simulink model "cloud9_powerTask"  (R2024b)
settings: Solver=VariableStepAuto  StartTime=0.0  StopTime=10.0  RelTol=1e-3
libraries: spsThreePhaseVIMeasurementLib x6, spsThreePhaseTransformerTwoWindingsLib x5, spsThreePhaseBreakerLib x4, spsThreePhaseSourceLib x3, spsThreePhaseParallelRLCBranchLib x1, sps_lib x1
settings Model: Creator=ASUS  LastModifiedBy=ASUS

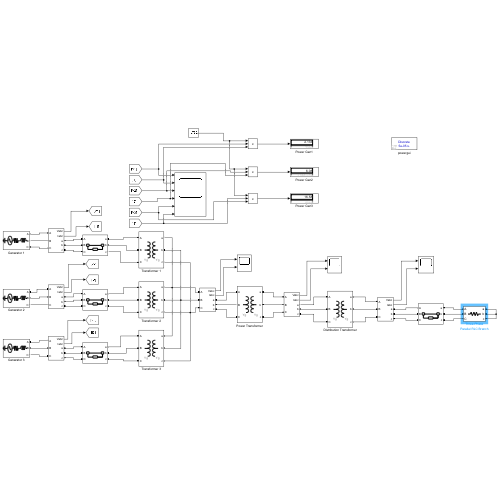
[thumbnail: Simulink's stored preview of the top-level diagram]
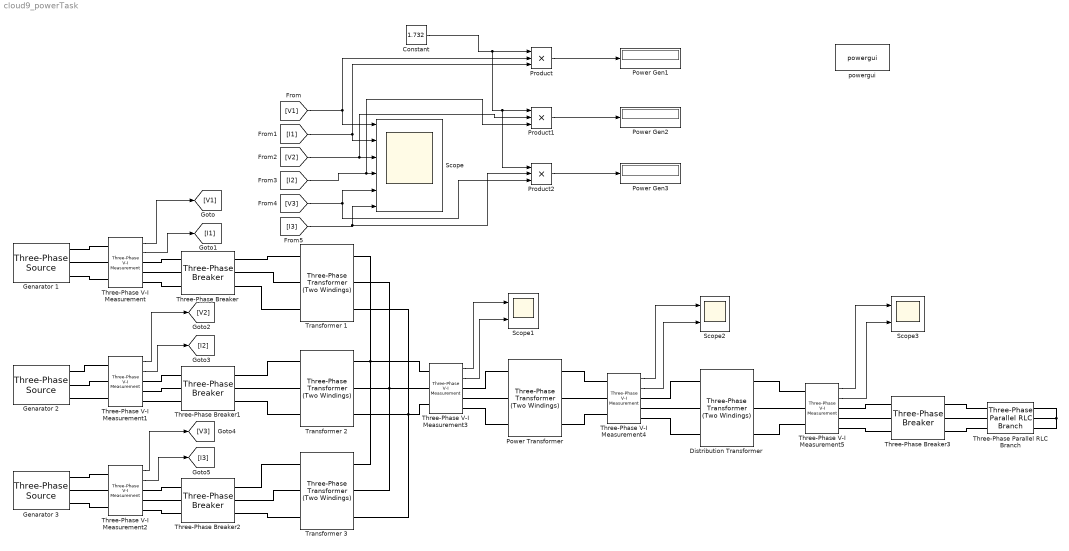
== system cloud9_powerTask ==
  Constant : Constant  Value=1.732
  Distribution Transformer : spsThreePhaseTransformerTwoWindingsLib/Three-Phase Transformer (Two Windings)  Winding1Connection=Yg  Winding2Connection=Yg  CoreType=Three single-phase transformers  SetSaturation=off  Hysteresis=off  DataFile='hysteresis'  SetInitialFlux=off  Measurements=None  UNITS=pu  NominalPower=[ 2e6 , 50 ]  Winding1=[ 11e3 , 0.002 , 0.08 ]  Winding2=[ 0.4e3 , 0.002 , 0.08 ]  Rm=500  Lm=500  L0=0.5  Saturation=[ 0,0 ; 0.0024,1.2 ; 1.0,1.52 ]  InitialFluxes=[ 0.8 , -0.8 , 0.7 ]  BreakLoop=off  DiscreteSolver=Trapezoidal iterative  DataType=off  TransfoNumber=1
  Genarator 1 : spsThreePhaseSourceLib/Three-Phase Source  InternalConnection=Yg  VoltagePhases=off  Voltage=11e3  PhaseAngle=0  Voltage_phases=[25e3 25e3 25e3]/sqrt(3)  PhaseAngles_phases=[0 -120 +120]  Frequency=50  NonIdealSource=on  SpecifyImpedance=off  Resistance=0.8929  Inductance=16.58e-3  ShortCircuitLevel=100e6  BaseVoltage=11e3  XRratio=7  BusType=PV  Pref=1000e3  Qref=0  Prefabc=[10e3, 10e3, 10e3]  Qrefabc=[0, 0, 0]  Qmin=-inf  Qmax=inf
  Genarator 2 : spsThreePhaseSourceLib/Three-Phase Source  InternalConnection=Yg  VoltagePhases=off  Voltage=12e3  PhaseAngle=0  Voltage_phases=[25e3 25e3 25e3]/sqrt(3)  PhaseAngles_phases=[0 -120 +120]  Frequency=50  NonIdealSource=on  SpecifyImpedance=off  Resistance=0.8929  Inductance=16.58e-3  ShortCircuitLevel=100e6  BaseVoltage=12e3  XRratio=7  BusType=PV  Pref=2000e3  Qref=0  Prefabc=[10e3, 10e3, 10e3]  Qrefabc=[0, 0, 0]  Qmin=-inf  Qmax=inf
  Genarator 3 : spsThreePhaseSourceLib/Three-Phase Source  InternalConnection=Yg  VoltagePhases=off  Voltage=10e3  PhaseAngle=0  Voltage_phases=[25e3 25e3 25e3]/sqrt(3)  PhaseAngles_phases=[0 -120 +120]  Frequency=50  NonIdealSource=on  SpecifyImpedance=off  Resistance=0.8929  Inductance=16.58e-3  ShortCircuitLevel=100e6  BaseVoltage=10e3  XRratio=7  BusType=PV  Pref=4000e3  Qref=0  Prefabc=[10e3, 10e3, 10e3]  Qrefabc=[0, 0, 0]  Qmin=-inf  Qmax=inf
  Power Gen1 : Display
  Power Gen2 : Display
  Power Gen3 : Display
  Power Transformer : spsThreePhaseTransformerTwoWindingsLib/Three-Phase Transformer (Two Windings)  Winding1Connection=Yg  Winding2Connection=Yg  CoreType=Three single-phase transformers  SetSaturation=off  Hysteresis=off  DataFile='hysteresis'  SetInitialFlux=off  Measurements=None  UNITS=pu  NominalPower=[ 7e6 , 50 ]  Winding1=[ 132e3 , 0.002 , 0.08 ]  Winding2=[ 11e3 , 0.002 , 0.08 ]  Rm=500  Lm=200  L0=0.5  Saturation=[ 0,0 ; 0.0024,1.2 ; 1.0,1.52 ]  InitialFluxes=[ 0.8 , -0.8 , 0.7 ]  BreakLoop=off  DiscreteSolver=Trapezoidal iterative  DataType=off  TransfoNumber=1
  Product : Product  Inputs=3
  Product1 : Product  Inputs=3
  Product2 : Product  Inputs=3
  Scope : Scope  NumInputPorts=6
  Scope1 : Scope  NumInputPorts=2
  Scope2 : Scope  NumInputPorts=2
  Scope3 : Scope  NumInputPorts=2
  Three-Phase Parallel RLC Branch : spsThreePhaseParallelRLCBranchLib/Three-Phase Parallel RLC Branch  LConnTagsString=A|B|C  RConnTagsString=A|B|C  BranchType=R  Resistance=7000000  Inductance=1e-3  Capacitance=1e-6  Measurements=None
  Three-Phase V-I Measurement{,1..5} (6 alike) : spsThreePhaseVIMeasurementLib/Three-Phase V-I Measurement  VoltageMeasurement=phase-to-ground  SetLabelV=off  LabelV=Vabc  Vpu=off  VpuLL=off  CurrentMeasurement=yes  SetLabelI=off  LabelI=Iabc  Ipu=off  Pbase=100e6  Vbase=500e3  OutputType=Complex  PhasorSimulation=off  PSBequivalent=0
  Three-Phase Breaker{,1..3} (4 alike) : spsThreePhaseBreakerLib/Three-Phase Breaker  InitialState=closed  SwitchA=on  SwitchB=on  SwitchC=on  SwitchTimes="[1/60  5/60]"  External=off  BreakerResistance=0.01  SnubberResistance=1e6  SnubberCapacitance=inf  Measurements=None
  Transformer 1 : spsThreePhaseTransformerTwoWindingsLib/Three-Phase Transformer (Two Windings)  Winding1Connection=Yg  Winding2Connection=Yg  CoreType=Three single-phase transformers  SetSaturation=off  Hysteresis=off  DataFile='hysteresis'  SetInitialFlux=off  Measurements=None  UNITS=pu  NominalPower=[ 1e6 , 50 ]  Winding1=[ 11e3 , 0.002 , 0.08 ]  Winding2=[ 132e3 , 0.002 , 0.08 ]  Rm=500  Lm=200  L0=0.5  Saturation=[ 0,0 ; 0.0024,1.2 ; 1.0,1.52 ]  InitialFluxes=[ 0.8 , -0.8 , 0.7 ]  BreakLoop=off  DiscreteSolver=Trapezoidal iterative  DataType=off  TransfoNumber=1
  Transformer 2 : spsThreePhaseTransformerTwoWindingsLib/Three-Phase Transformer (Two Windings)  Winding1Connection=Yg  Winding2Connection=Yg  CoreType=Three single-phase transformers  SetSaturation=off  Hysteresis=off  DataFile='hysteresis'  SetInitialFlux=off  Measurements=None  UNITS=pu  NominalPower=[ 2e6 , 50 ]  Winding1=[ 12e3 , 0.002 , 0.08 ]  Winding2=[ 132e3 , 0.002 , 0.08 ]  Rm=500  Lm=200  L0=0.5  Saturation=[ 0,0 ; 0.0024,1.2 ; 1.0,1.52 ]  InitialFluxes=[ 0.8 , -0.8 , 0.7 ]  BreakLoop=off  DiscreteSolver=Trapezoidal iterative  DataType=off  TransfoNumber=1
  Transformer 3 : spsThreePhaseTransformerTwoWindingsLib/Three-Phase Transformer (Two Windings)  Winding1Connection=Yg  Winding2Connection=Yg  CoreType=Three single-phase transformers  SetSaturation=off  Hysteresis=off  DataFile='hysteresis'  SetInitialFlux=off  Measurements=None  UNITS=pu  NominalPower=[ 4e6 , 50 ]  Winding1=[ 10e3 , 0.002 , 0.08 ]  Winding2=[ 132e3 , 0.002 , 0.08 ]  Rm=500  Lm=200  L0=0.5  Saturation=[ 0,0 ; 0.0024,1.2 ; 1.0,1.52 ]  InitialFluxes=[ 0.8 , -0.8 , 0.7 ]  BreakLoop=off  DiscreteSolver=Trapezoidal iterative  DataType=off  TransfoNumber=1
  powergui : sps_lib/powergui  Priority=1  SimulationMode=Discrete  SampleTime=50e-6  frequency=60  Iterations=50  frequencyindice=50  Pbase=100e6  ErrMax=1e-4  UnitsV=kV  UnitsW=MW  buscounter=0  FunctionMessages=off  echomessages=off  EnableUseOfTLC=off  CurrentSourceSwitches=off  DisableSnubberDevices=off  DisableRonSwitches=off  DisableVfSwitches=off  DisplayEquations=off  AutomaticDiscreteSolvers=off  SolverType=Tustin/Backward Euler (TBE)  Interpol=off  ExternalGateDelay=off  methode=off  Ts=100  x0status=blocks  SPID=on  SwTol=0  HookPort=off  NonlinearTolerance=1e-4  nMaxIteration=100  ContinueOnMaxIteration=off  RestoreLinks=warning  ResistiveCurrentMeasurement=off  Frange=[0:2:500]  Ylog=off  Xlog=on  ShowGrid=off  save=off  variable=ZData  structure=0  ZoomFFT=off  StartTime=0.0  cycles=1  DisplayStyle=1  fundamental=60  FreqAxis=off  MaxFrequency=1000  frequencyindicesteady=1  RmsSteady=1  display=off
  wires:
  Three-Phase V-I Measurement/1 -> [V1]
  Three-Phase V-I Measurement/2 -> [I1]
  Three-Phase V-I Measurement1/1 -> [V2]
  Three-Phase V-I Measurement1/2 -> [I2]
  Three-Phase V-I Measurement2/1 -> [V3]
  Three-Phase V-I Measurement2/2 -> [I3]
  [V1] -> Scope/1, Product/2
  [I1] -> Product/3, Scope/2
  [V2] -> Product1/2, Scope/3
  [I2] -> Product1/3, Scope/4
  [V3] -> Scope/5, Product2/3
  [I3] -> Product2/2, Scope/6
  Three-Phase V-I Measurement3/1 -> Scope1/1
  Three-Phase V-I Measurement3/2 -> Scope1/2
  Three-Phase V-I Measurement4/1 -> Scope2/1
  Three-Phase V-I Measurement4/2 -> Scope2/2
  Three-Phase V-I Measurement5/1 -> Scope3/1
  Three-Phase V-I Measurement5/2 -> Scope3/2
  Constant/1 -> Product2/1, Product1/1, Product/1
  Product/1 -> Power Gen1/1
  Product1/1 -> Power Gen2/1
  Product2/1 -> Power Gen3/1
  connections:
  Three-Phase Breaker/RConn1 -- Transformer 1/LConn1
  Three-Phase Breaker/RConn2 -- Transformer 1/LConn2
  Three-Phase Breaker/RConn3 -- Transformer 1/LConn3
  Three-Phase Breaker1/RConn1 -- Transformer 2/LConn1
  Three-Phase Breaker1/RConn2 -- Transformer 2/LConn2
  Three-Phase Breaker1/RConn3 -- Transformer 2/LConn3
  Three-Phase Breaker2/RConn1 -- Transformer 3/LConn1
  Three-Phase Breaker2/RConn2 -- Transformer 3/LConn2
  Three-Phase Breaker2/RConn3 -- Transformer 3/LConn3
  Genarator 1/RConn1 -- Three-Phase V-I Measurement/LConn1
  Genarator 1/RConn2 -- Three-Phase V-I Measurement/LConn2
  Genarator 1/RConn3 -- Three-Phase V-I Measurement/LConn3
  Genarator 2/RConn1 -- Three-Phase V-I Measurement1/LConn1
  Genarator 2/RConn2 -- Three-Phase V-I Measurement1/LConn2
  Genarator 2/RConn3 -- Three-Phase V-I Measurement1/LConn3
  Genarator 3/RConn1 -- Three-Phase V-I Measurement2/LConn1
  Genarator 3/RConn2 -- Three-Phase V-I Measurement2/LConn2
  Genarator 3/RConn3 -- Three-Phase V-I Measurement2/LConn3
  Three-Phase V-I Measurement/RConn1 -- Three-Phase Breaker/LConn1
  Three-Phase V-I Measurement/RConn2 -- Three-Phase Breaker/LConn2
  Three-Phase V-I Measurement/RConn3 -- Three-Phase Breaker/LConn3
  Three-Phase V-I Measurement1/RConn1 -- Three-Phase Breaker1/LConn1
  Three-Phase V-I Measurement1/RConn2 -- Three-Phase Breaker1/LConn2
  Three-Phase V-I Measurement1/RConn3 -- Three-Phase Breaker1/LConn3
  Three-Phase V-I Measurement2/RConn1 -- Three-Phase Breaker2/LConn1
  Three-Phase V-I Measurement2/RConn2 -- Three-Phase Breaker2/LConn2
  Three-Phase V-I Measurement2/RConn3 -- Three-Phase Breaker2/LConn3
  Three-Phase V-I Measurement3/LConn1 -- Transformer 3/RConn1 -- Transformer 1/RConn1 -- Transformer 2/RConn1
  Transformer 2/RConn2 -- Transformer 1/RConn2 -- Three-Phase V-I Measurement3/LConn2 -- Transformer 3/RConn2
  Transformer 2/RConn3 -- Transformer 1/RConn3 -- Three-Phase V-I Measurement3/LConn3 -- Transformer 3/RConn3
  Three-Phase V-I Measurement3/RConn1 -- Power Transformer/LConn1
  Three-Phase V-I Measurement3/RConn2 -- Power Transformer/LConn2
  Three-Phase V-I Measurement3/RConn3 -- Power Transformer/LConn3
  Power Transformer/RConn2 -- Three-Phase V-I Measurement4/LConn2
  Power Transformer/RConn3 -- Three-Phase V-I Measurement4/LConn3
  Power Transformer/RConn1 -- Three-Phase V-I Measurement4/LConn1
  Three-Phase V-I Measurement4/RConn1 -- Distribution Transformer/LConn1
  Three-Phase V-I Measurement4/RConn2 -- Distribution Transformer/LConn2
  Three-Phase V-I Measurement4/RConn3 -- Distribution Transformer/LConn3
  Distribution Transformer/RConn1 -- Three-Phase V-I Measurement5/LConn1
  Distribution Transformer/RConn2 -- Three-Phase V-I Measurement5/LConn2
  Distribution Transformer/RConn3 -- Three-Phase V-I Measurement5/LConn3
  Three-Phase V-I Measurement5/RConn1 -- Three-Phase Breaker3/LConn1
  Three-Phase V-I Measurement5/RConn2 -- Three-Phase Breaker3/LConn2
  Three-Phase V-I Measurement5/RConn3 -- Three-Phase Breaker3/LConn3
  Three-Phase Breaker3/RConn1 -- Three-Phase Parallel RLC Branch/LConn1
  Three-Phase Breaker3/RConn2 -- Three-Phase Parallel RLC Branch/LConn2
  Three-Phase Breaker3/RConn3 -- Three-Phase Parallel RLC Branch/LConn3
  Three-Phase Parallel RLC Branch/RConn1 -- Three-Phase Parallel RLC Branch/RConn2 -- Three-Phase Parallel RLC Branch/RConn3
